simulink model "Rejz3"  (R2021a)
settings: Solver=VariableStepAuto  StartTime=0.0  StopTime=30.0  RelTol=1e-3
values from neighbouring files (symbols this model uses):
  A = [-1/T1 0 0; 1/T2 -1/T2 0; 0 A1/T3 -1/T3]    [maj11.m]
  B = [1/T1; 0; 0]    [maj11.m]
  C = [0 0 1]    [maj11.m]
  Fh = Ah - Gh *Ch    [maj11.m]
  Gh = Ght'    [maj11.m]
  Hh = Bh    [maj11.m]
  K = acker(A, B, [s1 s2 scinf])    [maj11.m]
  Nu = Nxu( end)    [maj11.m]
  Nx = Nxu(1:3)    [maj11.m]
settings Model: Creator=Peti  LastModifiedBy=Peti

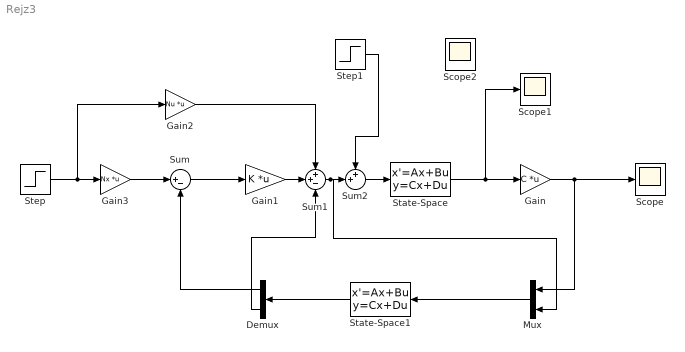
== system Rejz3 ==
  Demux : Demux  Outputs=[3,1]
  Gain : Gain  Gain=C  Multiplication=Matrix(K*u)
  Gain1 : Gain  Gain=K  Multiplication=Matrix(K*u)
  Gain2 : Gain  Gain=Nu  Multiplication=Matrix(K*u)
  Gain3 : Gain  Gain=Nx  Multiplication=Matrix(K*u)
  Mux : Mux  Inputs=2
  Scope : Scope
  Scope1 : Scope
  Scope2 : Scope
  State-Space : StateSpace  A=A  B=B  C=eye(3)  D=zeros(3, 1)  InitialCondition=[0 0 0 ]
  State-Space1 : StateSpace  A=Fh  B=[Gh Hh]  C=eye(4)  D=zeros(4,2)  InitialCondition=[0 0 0 0]
  Step : Step  SampleTime=0
  Step1 : Step  Time=15  After=5  SampleTime=0
  Sum : Sum  Inputs=|+-
  Sum1 : Sum  Inputs=++-
  Sum2 : Sum  Inputs=++|
  wires:
  State-Space/1 -> Scope1/1, Gain/1
  Gain/1 -> Mux/1, Scope/1
  Sum/1 -> Gain1/1
  Step/1 -> Gain2/1, Gain3/1
  Gain3/1 -> Sum/1
  Sum1/1 -> Mux/2, Sum2/2
  Gain1/1 -> Sum1/2
  Gain2/1 -> Sum1/1
  Mux/1 -> State-Space1/1
  State-Space1/1 -> Demux/1
  Demux/1 -> Sum/2
  Demux/2 -> Sum1/3
  Sum2/1 -> State-Space/1
  Step1/1 -> Sum2/1
